simulink model "pendbasic_plotting"  (Simulink 7.9)
settings: Solver=ode45  StartTime=0.0  StopTime=1000  RelTol=1e-3
values from neighbouring files (symbols this model uses):
  h = 0.01    [pendinit.m]
  k1 = 0.058    [pendinit.m]
  k2 = 0.68    [pendinit.m]
  k360 = 0.3091    [pendinit.m]
  k4r = 2.56    [pendinit.m]
  k5r = 2.0    (= 2)    [pendinit.m]
  kdot360 = 3.76    [pendinit.m]
  ku = 1.40    (= 1.4)    [pendinit.m]
  Lnopos = dlqr(Afd,Bfd,Q,R)    [pendinit.m]
  Lpos = dlqr(Afd,Bfd,Q,R)    [pendinit.m]
  offs1 = 0.7792-0.035/k1    (= 0.175751724138)    [pendinit.m]
  offs2 = 0    [pendinit.m]
  offs360 = 5.1763    [pendinit.m]
  offs4r = 0    [pendinit.m]
  offs5r = 0.0708+0.16/k5r    (= 0.1508)    [pendinit.m]
  offsdot360 = -0.022    [pendinit.m]
settings Model: Creator=tfy12aja  LastModifiedBy=tfy12aja

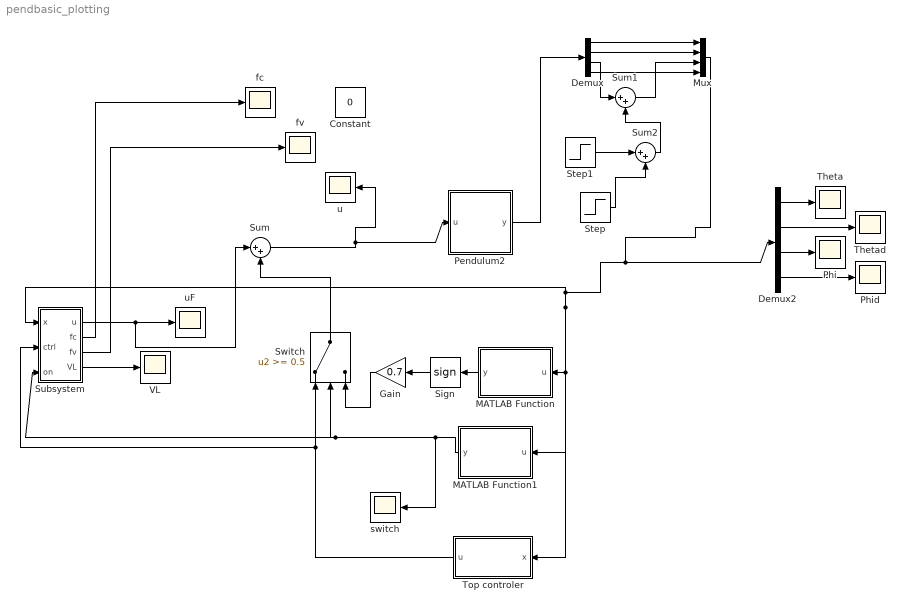
== system pendbasic_plotting ==
  Constant : Constant  Value=0
  Demux : Demux
  Demux2 : Demux
  Gain : Gain  Gain=0.7
  MATLAB Function : MATLAB Function  TreatAsAtomicUnit=on
  MATLAB Function1 : MATLAB Function  TreatAsAtomicUnit=on
  Mux : Mux
  Pendulum2 : Subsystem
      mask Display: disp('Hardware\n Lab 2 Nonlin')
  Phi : Scope
      settings: TimeRange=25  YMin=-0.35  YMax=0.4  SaveName=ScopeData7
  Phid : Scope
      settings: YMin=-0.7  YMax=1.5  SaveName=ScopeData8
  Sign : Signum
  Step : Step  Time=25  After=-2  SampleTime=0
  Step1 : Step  Time=15  SampleTime=0
  Subsystem : Subsystem
  Sum : Sum  Inputs=|++
  Sum1 : Sum  Inputs=|++
  Sum2 : Sum  Inputs=|++
  Switch : Switch  Threshold=0.5
  Theta : Scope
      settings: YMin=-0.0175  YMax=0.015  SaveName=ScopeData9
  Thetad : Scope
      settings: YMin=-0.15  YMax=0.125  SaveName=ScopeData10
  Top controler : Subsystem
  VL : Scope
      settings: YMin=-850  YMax=100  SaveName=ScopeData6
  fc : Scope
      settings: YMin=0.54  YMax=0.58  SaveName=ScopeData4
  fv : Scope
      settings: YMin=-0.06  YMax=-0.0075  SaveName=ScopeData5
  switch : Scope
      settings: YMin=-1  YMax=1.25
  u : Scope
      settings: YMin=-1  YMax=1.25  SaveName=ScopeData11
  uF : Scope
      settings: YMin=-4.5  YMax=2  SaveName=ScopeData12
  wires:
  Demux2/2 -> Thetad/1
  Demux2/3 -> Phi/1
  Demux2/4 -> Phid/1
  Demux2/1 -> Theta/1
  Mux/1 -> Demux2/1, MATLAB Function/1(u), MATLAB Function1/1(u), Top controler/1(x), Subsystem/1(x)
  MATLAB Function/1(y) -> Sign/1
  Sign/1 -> Gain/1
  MATLAB Function1/1(y) -> switch/1, Switch/2, Subsystem/3(on)
  Gain/1 -> Switch/3
  Subsystem/3(fv) -> fv/1
  Subsystem/4(VL) -> VL/1
  Subsystem/2(fc) -> fc/1
  Subsystem/1(u) -> uF/1, Sum/1
  Top controler/1(u) -> Switch/1, Subsystem/2(ctrl)
  Switch/1 -> Sum/2
  Sum/1 -> u/1, Pendulum2/1(u)
  Demux/4 -> Mux/4
  Demux/2 -> Mux/2
  Demux/1 -> Mux/1
  Demux/3 -> Sum1/1
  Sum1/1 -> Mux/3
  Sum2/1 -> Sum1/2
  Step/1 -> Sum2/2
  Step1/1 -> Sum2/1
  Pendulum2/1(y) -> Demux/1

== system pendbasic_plotting/Pendulum2 ==
  u : Inport
  Hardware : Subsystem
  Safety net (switch off) : Subsystem
  Terminator : Terminator
  y : Outport  InitialOutput=0
  tag scope: u=global
  wires:
  [u] -> Terminator/1
  u/1 -> Safety net (switch off)/1(u_in)
  Safety net (switch off)/1(u_out) -> Hardware/1(u), [u]
  Hardware/1(y) -> y/1

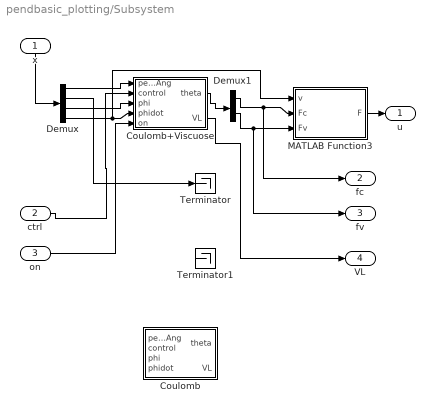
== system pendbasic_plotting/Subsystem ==
  x : Inport
  ctrl : Inport  Port=2
  on : Inport  Port=3
  Coulomb : MATLAB Function  TreatAsAtomicUnit=on
  Coulomb+Viscuose : MATLAB Function  TreatAsAtomicUnit=on
  Demux : Demux
  Demux1 : Demux  Outputs=2
  MATLAB Function3 : MATLAB Function  TreatAsAtomicUnit=on
  Terminator : Terminator
  Terminator1 : Terminator
  u : Outport
  fc : Outport  Port=2
  fv : Outport  Port=3
  VL : Outport  Port=4
  wires:
  Coulomb+Viscuose/1(theta) -> Demux1/1
  x/1 -> Demux/1
  Demux1/1 -> fc/1, MATLAB Function3/2(Fc)
  Demux1/2 -> fv/1, MATLAB Function3/3(Fv)
  MATLAB Function3/1(F) -> u/1
  Demux/1 -> Coulomb+Viscuose/1(pendAng)
  Demux/4 -> MATLAB Function3/1(v), Coulomb+Viscuose/4(phidot)
  Demux/2 -> Terminator/1
  Demux/3 -> Coulomb+Viscuose/3(phi)
  ctrl/1 -> Coulomb+Viscuose/2(control)
  Coulomb+Viscuose/2(VL) -> VL/1
  on/1 -> Coulomb+Viscuose/5(on)

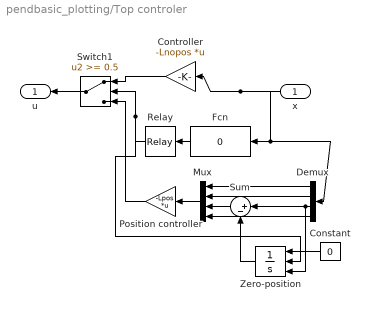
== system pendbasic_plotting/Top controler ==
  x : Inport
  Constant : Constant  Value=0
  Controller : Gain  Gain=-Lnopos  Multiplication=Matrix(K*u)  SaturateOnIntegerOverflow=on  OutDataTypeStr=Inherit: Same as input  ParamDataTypeStr=Inherit: Same as input
  Demux : Demux
  Fcn : Fcn  Expr=0
  Mux : Mux
  Position controller : Gain  Gain=-Lpos  Multiplication=Matrix(K*u)  SaturateOnIntegerOverflow=on  OutDataTypeStr=Inherit: Same as input  ParamDataTypeStr=Inherit: Same as input
  Relay : Relay  OnSwitchValue=4  OffSwitchValue=3.9
  Sum : Sum  Inputs=|+-  SaturateOnIntegerOverflow=on  InputSameDT=on  OutDataTypeStr=Inherit: Same as first input
  Switch1 : Switch  Threshold=0.5  SaturateOnIntegerOverflow=on  InputSameDT=on
  Zero-position : Integrator  ExternalReset=falling  InitialConditionSource=external
  u : Outport
  wires:
  Switch1/1 -> u/1
  Sum/1 -> Mux/3
  Zero-position/1 -> Sum/2
  Fcn/1 -> Relay/1
  Constant/1 -> Zero-position/1
  Demux/3 -> Sum/1, Zero-position/3
  Demux/4 -> Mux/4
  Demux/2 -> Mux/2
  Demux/1 -> Mux/1
  Mux/1 -> Position controller/1
  Controller/1 -> Switch1/1
  Relay/1 -> Zero-position/2, Switch1/2
  Position controller/1 -> Switch1/3
  x/1 -> Demux/1, Fcn/1, Controller/1

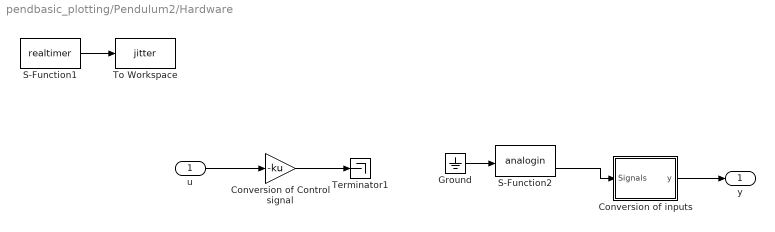
== system pendbasic_plotting/Pendulum2/Hardware ==
  u : Inport
  Conversion of Control signal : Gain  Gain=-ku  SaturateOnIntegerOverflow=on  OutDataTypeStr=Inherit: Same as input  ParamDataTypeStr=Inherit: Same as input
  Conversion of inputs : Subsystem
  Ground : Ground
  S-Function1 : S-Function  FunctionName=realtimer  Parameters=h  EnableBusSupport=off
  S-Function2 : S-Function  FunctionName=analogin  Parameters=h [0 0 1 1 2 2 3 3 4 4 5 5 6 6 7 7]  EnableBusSupport=off
  Terminator1 : Terminator
  To Workspace : ToWorkspace  VariableName=jitter  SampleTime=-1
  y : Outport
  wires:
  Conversion of inputs/1(y) -> y/1
  S-Function1/1 -> To Workspace/1
  Conversion of Control signal/1 -> Terminator1/1
  S-Function2/2 -> Conversion of inputs/1(Signals)
  Ground/1 -> S-Function2/1
  u/1 -> Conversion of Control signal/1

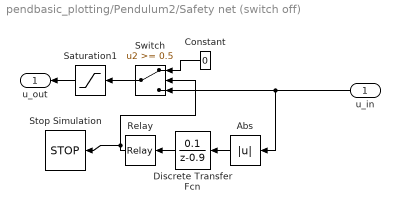
== system pendbasic_plotting/Pendulum2/Safety net (switch off) ==
  u_in : Inport
  Abs : Abs  SaturateOnIntegerOverflow=on
  Constant : Constant  Value=0
  Discrete Transfer Fcn : DiscreteTransferFcn  Numerator=[0.1]  Denominator=[1 -0.9]  SampleTime=h
  Relay : Relay  OnSwitchValue=3  OffSwitchValue=2
  Saturation1 : Saturate  UpperLimit=2  LowerLimit=-2
  Stop Simulation : Stop
  Switch : Switch  Threshold=0.5  SaturateOnIntegerOverflow=on  InputSameDT=on
  u_out : Outport
  wires:
  u_in/1 -> Abs/1, Switch/3
  Saturation1/1 -> u_out/1
  Switch/1 -> Saturation1/1
  Abs/1 -> Discrete Transfer Fcn/1
  Constant/1 -> Switch/1
  Relay/1 -> Switch/2, Stop Simulation/1
  Discrete Transfer Fcn/1 -> Relay/1

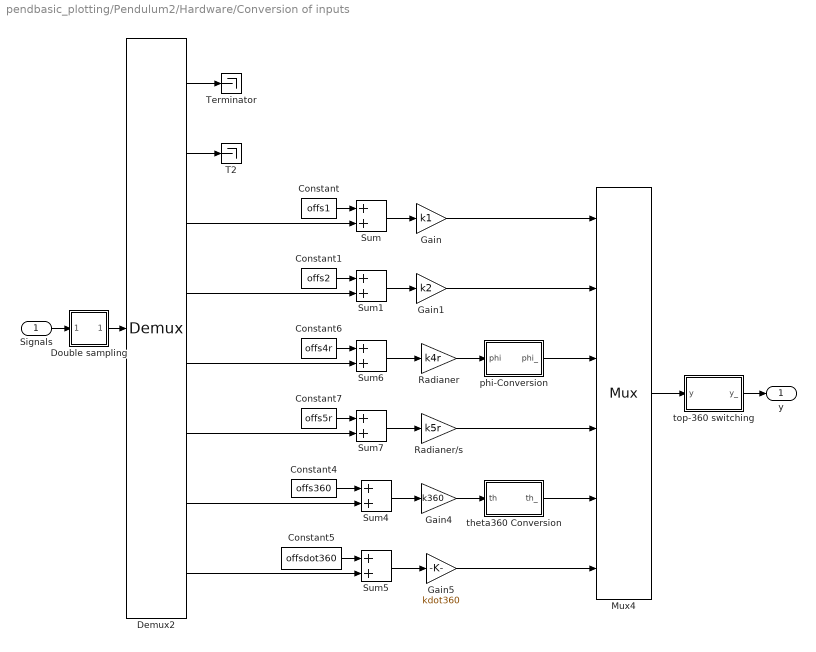
== system pendbasic_plotting/Pendulum2/Hardware/Conversion of inputs ==
  Signals : Inport
  Constant : Constant  Value=offs1
  Constant1 : Constant  Value=offs2
  Constant4 : Constant  Value=offs360
  Constant5 : Constant  Value=offsdot360
  Constant6 : Constant  Value=offs4r
  Constant7 : Constant  Value=offs5r
  Demux2 : Demux  Outputs=8
  Double sampling : Subsystem
  Gain : Gain  Gain=k1  SaturateOnIntegerOverflow=on  OutDataTypeStr=Inherit: Same as input  ParamDataTypeStr=Inherit: Same as input
  Gain1 : Gain  Gain=k2  SaturateOnIntegerOverflow=on  OutDataTypeStr=Inherit: Same as input  ParamDataTypeStr=Inherit: Same as input
  Gain4 : Gain  Gain=k360  SaturateOnIntegerOverflow=on  OutDataTypeStr=Inherit: Same as input  ParamDataTypeStr=Inherit: Same as input
  Gain5 : Gain  Gain=kdot360  SaturateOnIntegerOverflow=on  OutDataTypeStr=Inherit: Same as input  ParamDataTypeStr=Inherit: Same as input
  Mux4 : Mux  Inputs=6
  Radianer : Gain  Gain=k4r  SaturateOnIntegerOverflow=on  OutDataTypeStr=Inherit: Same as input  ParamDataTypeStr=Inherit: Same as input
  Radianer/s : Gain  Gain=k5r  SaturateOnIntegerOverflow=on  OutDataTypeStr=Inherit: Same as input  ParamDataTypeStr=Inherit: Same as input
  Sum{,1,4..7} (6 alike) : Sum  SaturateOnIntegerOverflow=on  InputSameDT=on  OutDataTypeStr=Inherit: Same as first input
  T2 : Terminator
  Terminator : Terminator
  phi-Conversion : Subsystem
  theta360 Conversion : Subsystem
  top-360 switching : Subsystem
  y : Outport  InitialOutput=0
  wires:
  Gain1/1 -> Mux4/2
  Demux2/8 -> Sum5/2
  Demux2/7 -> Sum4/2
  Demux2/4 -> Sum1/2
  Demux2/3 -> Sum/2
  Gain/1 -> Mux4/1
  Gain5/1 -> Mux4/6
  Gain4/1 -> theta360 Conversion/1(th)
  Double sampling/1(Out1) -> Demux2/1
  Signals/1 -> Double sampling/1(In1)
  theta360 Conversion/1(th_) -> Mux4/5
  Radianer/s/1 -> Mux4/4
  phi-Conversion/1(phi_) -> Mux4/3
  Demux2/6 -> Sum7/2
  Demux2/5 -> Sum6/2
  Constant4/1 -> Sum4/1
  top-360 switching/1(y_) -> y/1
  Mux4/1 -> top-360 switching/1(y)
  Constant7/1 -> Sum7/1
  Sum7/1 -> Radianer/s/1
  Radianer/1 -> phi-Conversion/1(phi)
  Constant6/1 -> Sum6/1
  Sum6/1 -> Radianer/1
  Constant5/1 -> Sum5/1
  Sum5/1 -> Gain5/1
  Sum4/1 -> Gain4/1
  Constant1/1 -> Sum1/1
  Sum1/1 -> Gain1/1
  Constant/1 -> Sum/1
  Sum/1 -> Gain/1
  Demux2/1 -> Terminator/1
  Demux2/2 -> T2/1

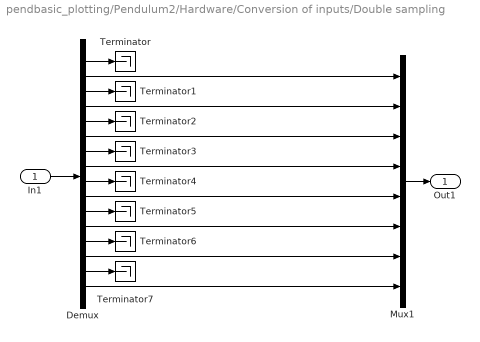
== system pendbasic_plotting/Pendulum2/Hardware/Conversion of inputs/Double sampling ==
  In1 : Inport
  Demux : Demux  Outputs=16
  Mux1 : Mux  Inputs=8
  Terminator{,1..7} (8 alike) : Terminator
  Out1 : Outport
  wires:
  Demux/16 -> Mux1/8
  Demux/14 -> Mux1/7
  Demux/12 -> Mux1/6
  Demux/10 -> Mux1/5
  Demux/8 -> Mux1/4
  Demux/6 -> Mux1/3
  Demux/4 -> Mux1/2
  Mux1/1 -> Out1/1
  Demux/2 -> Mux1/1
  In1/1 -> Demux/1
  Demux/1 -> Terminator/1
  Demux/3 -> Terminator1/1
  Demux/5 -> Terminator2/1
  Demux/15 -> Terminator7/1
  Demux/13 -> Terminator6/1
  Demux/11 -> Terminator5/1
  Demux/9 -> Terminator4/1
  Demux/7 -> Terminator3/1

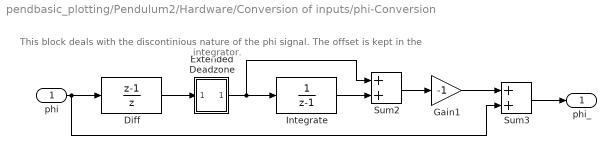
== system pendbasic_plotting/Pendulum2/Hardware/Conversion of inputs/phi-Conversion ==
  note: This block deals with the discontinious nature
      | of the phi signal. The offset is kept in the integrator.
  phi : Inport
  Diff : DiscreteTransferFcn  Numerator=[1 -1]  Denominator=[1 0]  SampleTime=h
  Extended Deadzone : Subsystem  mask{vg=1, dv=0.5}
      mask prompts: vg "Gain"; dv "Deadzone width"
      mask init:
      | v_gain=vg;
      | d_v=dv;
      mask Display:
      | plot([-1 0 0], [0 0 1], [0 0 1],[-1 0 0]);
      | plot([0.5 0.5 1],[0 0.5 1],[-0.5 -0.5 -1],[0 -0.5 -1]);
  Gain1 : Gain  Gain=-1  SaturateOnIntegerOverflow=on  OutDataTypeStr=Inherit: Same as input  ParamDataTypeStr=Inherit: Same as input
  Integrate : DiscreteTransferFcn  Denominator=[1 -1]  SampleTime=h
  Sum2 : Sum  SaturateOnIntegerOverflow=on  InputSameDT=on  OutDataTypeStr=Inherit: Same as first input
  Sum3 : Sum  SaturateOnIntegerOverflow=on  InputSameDT=on  OutDataTypeStr=Inherit: Same as first input
  phi_ : Outport
  wires:
  Diff/1 -> Extended Deadzone/1(In1)
  Sum3/1 -> phi_/1
  Extended Deadzone/1(Out1) -> Sum2/1, Integrate/1
  Integrate/1 -> Sum2/2
  Gain1/1 -> Sum3/1
  phi/1 -> Sum3/2, Diff/1
  Sum2/1 -> Gain1/1

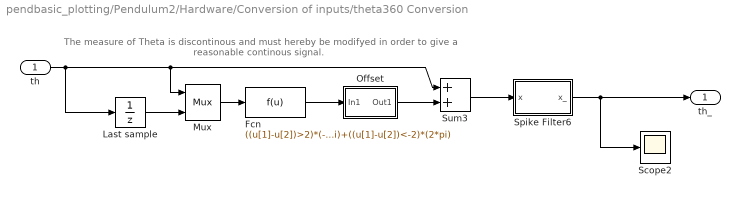
== system pendbasic_plotting/Pendulum2/Hardware/Conversion of inputs/theta360 Conversion ==
  note: The measure of Theta is discontinous and must hereby
      | be modifyed in order to give a reasonable continous signal.
  th : Inport
  Fcn : Fcn  Expr=((u[1]-u[2])>2)*(-2*pi)+((u[1]-u[2])<-2)*(2*pi)
  Last sample : UnitDelay  SampleTime=h
  Mux : Mux  Inputs=2
  Offset : Subsystem
  Scope2 : Scope
      settings: TimeRange=25  YMin=-0.4  YMax=0.05
  Spike Filter6 : Subsystem
  Sum3 : Sum  SaturateOnIntegerOverflow=on  InputSameDT=on  OutDataTypeStr=Inherit: Same as first input
  th_ : Outport
  wires:
  Spike Filter6/1(x_) -> Scope2/1, th_/1
  Sum3/1 -> Spike Filter6/1(x)
  Offset/1(Out1) -> Sum3/2
  Fcn/1 -> Offset/1(In1)
  Last sample/1 -> Mux/2
  th/1 -> Sum3/1, Mux/1, Last sample/1
  Mux/1 -> Fcn/1

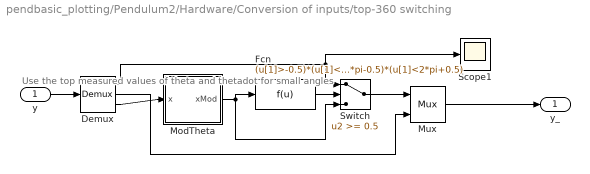
== system pendbasic_plotting/Pendulum2/Hardware/Conversion of inputs/top-360 switching ==
  note: Use the top measured values of
      | theta and thetadot for small angles
  y : Inport
  Demux : Demux  Outputs=[2 2 2]
  Fcn : Fcn  Expr=(u[1]>-0.5)*(u[1]<0.5)+(u[1]>2*pi-0.5)*(u[1]<2*pi+0.5)
  ModTheta : Subsystem
  Mux : Mux  Inputs=2
  Scope1 : Scope
      settings: YMin=-4  YMax=7  SaveName=ScopeData3
  Switch : Switch  Threshold=0.5  SaturateOnIntegerOverflow=on  InputSameDT=on
  y_ : Outport
  wires:
  Mux/1 -> y_/1
  Fcn/1 -> Switch/2
  Demux/1 -> Switch/1, Scope1/1
  Demux/2 -> Mux/2
  y/1 -> Demux/1
  Demux/3 -> ModTheta/1(x)
  ModTheta/1(xMod) -> Switch/3, Fcn/1
  Switch/1 -> Mux/1

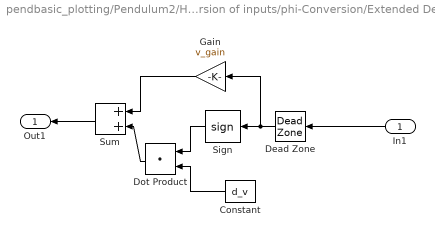
== system pendbasic_plotting/Pendulum2/Hardware/Conversion of inputs/phi-Conversion/Extended Deadzone ==
  In1 : Inport
  Constant : Constant  Value=d_v
  Dead Zone : DeadZone  LowerValue=-d_v  UpperValue=d_v  SaturateOnIntegerOverflow=on
  Dot Product : DotProduct  InputSameDT=on  OutDataTypeStr=Inherit: Inherit via internal rule
  Gain : Gain  Gain=v_gain  SaturateOnIntegerOverflow=on  OutDataTypeStr=Inherit: Same as input  ParamDataTypeStr=Inherit: Same as input
  Sign : Signum
  Sum : Sum  SaturateOnIntegerOverflow=on  InputSameDT=on  OutDataTypeStr=Inherit: Same as first input
  Out1 : Outport  InitialOutput=0
  wires:
  Gain/1 -> Sum/1
  In1/1 -> Dead Zone/1
  Sign/1 -> Dot Product/1
  Dead Zone/1 -> Gain/1, Sign/1
  Constant/1 -> Dot Product/2
  Dot Product/1 -> Sum/2
  Sum/1 -> Out1/1

== system pendbasic_plotting/Pendulum2/Hardware/Conversion of inputs/theta360 Conversion/Offset ==
  note: Make sure only one
      | trig per lap.
  In1 : Inport
  Fcn : Fcn  Expr=(abs(u[1]+u[2])>8)*0+(abs(u[1]+u[2])<8)*u[1]
  Integrate : DiscreteTransferFcn  Denominator=[1 -1]  SampleTime=h
  Last offset : UnitDelay  SampleTime=h
  Mux : Mux  Inputs=2
  Out1 : Outport  InitialOutput=0
  wires:
  Integrate/1 -> Out1/1
  Fcn/1 -> Integrate/1
  Last offset/1 -> Mux/2
  In1/1 -> Last offset/1, Mux/1
  Mux/1 -> Fcn/1

== system pendbasic_plotting/Pendulum2/Hardware/Conversion of inputs/theta360 Conversion/Spike Filter6 ==
  x : Inport
  Fcn : Fcn  Expr=(abs(u[1]-u[2])<0.5)*u[1]+(abs(u[1]-u[2])>0.5)*u[3]
  Last Chosen : UnitDelay  SampleTime=h
  Last sample : UnitDelay  SampleTime=h
  Mux : Mux  Inputs=3
  Scope1 : Scope
      settings: YMin=0  YMax=11
  Scope2 : Scope
      settings: YMin=9  YMax=9.9
  x_ : Outport
  wires:
  Mux/1 -> Scope2/1, Fcn/1
  Fcn/1 -> Last Chosen/1, Scope1/1, x_/1
  x/1 -> Mux/1, Last sample/1
  Last sample/1 -> Mux/2
  Last Chosen/1 -> Mux/3

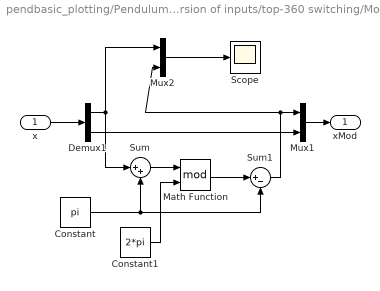
== system pendbasic_plotting/Pendulum2/Hardware/Conversion of inputs/top-360 switching/ModTheta ==
  x : Inport
  Constant : Constant  Value=pi
  Constant1 : Constant  Value=2*pi
  Demux1 : Demux  Outputs=2
  Math Function : Math  Operator=mod  SaturateOnIntegerOverflow=on
  Mux1 : Mux  Inputs=2
  Mux2 : Mux  Inputs=2
  Scope : Scope
      settings: YMin=-4  YMax=7  SaveName=ScopeData2
  Sum : Sum  Inputs=|++
  Sum1 : Sum  Inputs=|+-
  xMod : Outport
  wires:
  Demux1/1 -> Mux2/1, Sum/1
  Mux2/1 -> Scope/1
  Constant/1 -> Sum/2, Sum1/2
  Demux1/2 -> Mux1/2
  Sum/1 -> Math Function/1
  Constant1/1 -> Math Function/2
  Math Function/1 -> Sum1/1
  Sum1/1 -> Mux1/1, Mux2/2
  x/1 -> Demux1/1
  Mux1/1 -> xMod/1

== matlab function MATLAB Function1 ==
  data: u input double; y output double
function y= fcn(u)
%#codegen
ar=sqrt(0.62^2+9.4^2);
ar=ar*0.2;
br=sqrt(0.19^2+2.5^2);
br=br*0.2;
alfar=atan(9.4/0.62);
X = u(1);
Y = u(2);

term1 = X*cos(alfar)+Y*sin(alfar);
term2 = -X*sin(alfar) + Y*cos(alfar);
y = (term1^2/ar^2 + term2^2/br^2) < 1.5;
%y2 = ((term1^2/ar^2 + term2^2/br^2) < 0.2) && (abs(X)>0.0000005) && (abs(Y)>0.006);

%y = abs(u(1)) + abs(u(2)) < 0.8;

== matlab function MATLAB Function ==
  data: u input double; y output double
function y = fcn(u)
%#codegen
omega0 =  7;%2*pi*0.9002;
y = cos(u(1))*u(2)*(cos(u(1))-1+u(2).^2/2/omega0^2);
%y = 0;

== matlab function Subsystem/Coulomb ==
  data: pendAng input double; theta output double; control input double; phi input double; phidot input double; VL output double
function [theta,VL]   = RLS(pendAng,control,phi,phidot)
%RLS Summary of this function goes here
%   Detailed explanation goes here
    persistent P_old;
    persistent theta_old;
    persistent regressor;
    persistent pendAng_old;
    persistent control_old;
    persistent phi_old;
    persistent phidot_old;
    pfc=1000;
    fcGuess=0.134;
    
if(isempty(P_old))
        P_old=pfc;
        theta_old = fcGuess;
        regressor = 0;
        pendAng_old = 0;
        control_old = 0;
        phi_old=0;
        phidot_old = 0;
        regressor_old = [0 0]';
end
VL = 0;
if(control~=1337) 
    P_old = P_old - (P_old*regressor*regressor' *P_old)/(1+regressor'*P_old*regressor);
    VL =(phidot+0.0059*pendAng_old-1.9125*control_old-phidot_old)/(-1.9125);
    epsilon = VL - regressor'*theta_old;
    theta_old = theta_old + P_old*regressor.*epsilon;
    regressor = sign(phidot)';
    pendAng_old = pendAng;
    control_old = control;
    phi_old = phi;
    phidot_old = phidot;
end
theta = [theta_old 0];

end

== matlab function Subsystem/MATLAB Function3 ==
  data: v input double; F output double; Fc input double; Fv input double
function F = fcn(v,Fc,Fv)
%persistent F_old
%if isempty(F_old)
%   F_old = 0;
%end

F = Fc*sign(v)+Fv*v;
%F_old = F;
end

== matlab function Subsystem/Coulomb+Viscuose ==
  data: pendAng input double; theta output double; control input double; phi input double; phidot input double; VL output double; on input double
function [theta,VL]   = RLS(pendAng,control,phi,phidot,on)
%RLS Summary of this function goes here
%   Detailed explanation goes here
    persistent P_old;
    persistent theta_old;
%    persistent regressor;
    persistent pendAng_old;
    persistent control_old;
    persistent phi_old;
    persistent phidot_old;
    pfc=1000;
    pfv=1000;
    fcGuess=0.134;
    fvGuess=0.02;
    lambda = 1;
if(isempty(P_old))
        P_old=[pfc 0;0 pfv];
        theta_old = [fcGuess fvGuess]';
%        regressor = [0 0]';
        pendAng_old = 0;
        control_old = 0;
        phi_old=0;
        phidot_old = 0;
end
if on
    regressor = [sign(phidot) phidot]';
    P_old = 1/lambda*(P_old - (P_old*regressor*regressor' *P_old)/(lambda+regressor'*P_old*regressor));
    VL =(phidot+0.0059*pendAng_old-1.9125*control_old-phidot_old)/(-1.9125);
    epsilon = VL - regressor'*theta_old;
    theta_old = theta_old + P_old*regressor.*epsilon;
    pendAng_old = pendAng;
    control_old = control;
    phidot_old = phidot;
    phi_old = phi;
    theta = theta_old;
else
    theta = [0 0]';
    VL = 0;
end
end
